simulink model "Bdot"  (R2023b)
settings: Solver=VariableStepAuto  StartTime=0.0  StopTime=2.647E4  FixedStep=1  MaxStep=100  RelTol=1e-3
model workspace (MAT data in the model file):
  Inertia = [0.0088  0  0; 0  0.0088  0; 0  0  0.004]
  M = 0.9
  T = 5580
libraries: matrix_library x2, shared6dof x1, simulink x1, aerolibanim x1
settings Model: Creator=bogas  LastModifiedBy=bogas

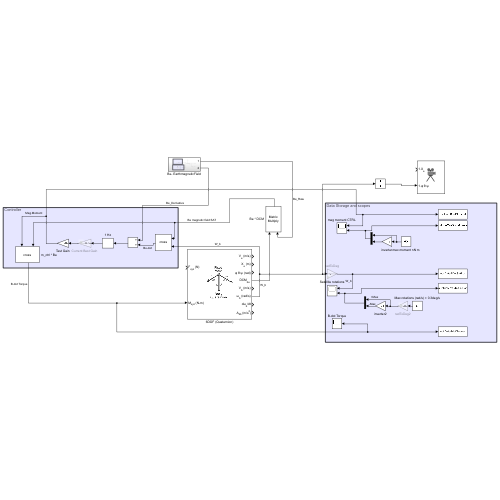
[thumbnail: Simulink's stored preview of the top-level diagram]
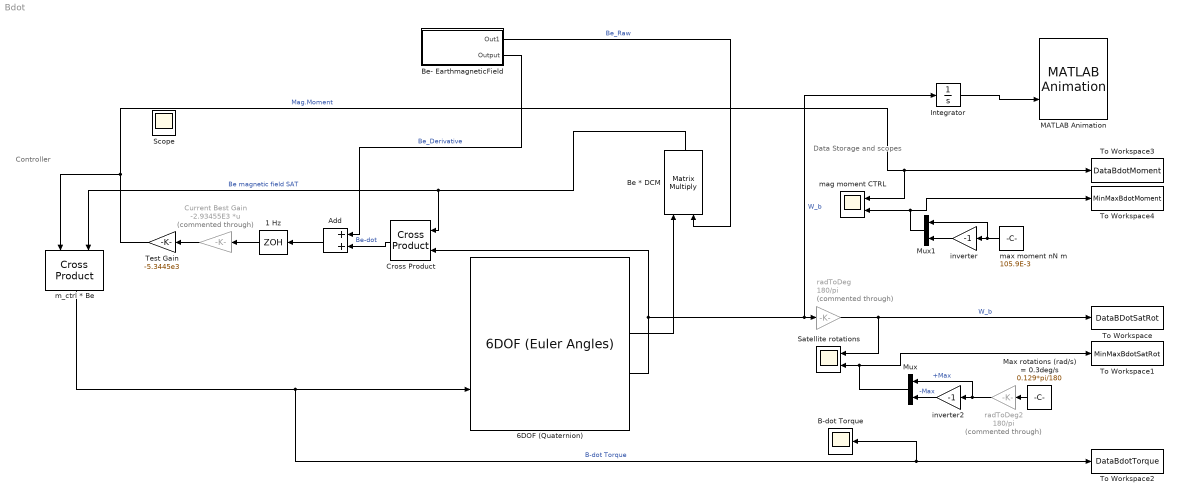
== system Bdot ==
  note: Controller
  note: Data Storage and scopes
  1 Hz : ZeroOrderHold
  6DOF (Quaternion) : shared6dof/6DOF (Euler Angles)  units=Metric (MKS)  mtype=Fixed  rep=Quaternion  xme_0=[0 0 0]  Vm_0=[0 0 0]  eul_0=[0 0 0]  pm_0=0.1745*[1,1,1]  mass_0=M  mass_e=0.5  mass_f=2.0  inertia=Inertia  inertia_e=eye(3)  inertia_f=2*eye(3)  k_quat=1.0  vre_flag=on  abi_flag=off  aMode=0  xme_statename=''  Vm_statename=''  eul_statename=''  quat_statename=''  pm_statename=''  mass_statename=''
      settings: LibrarySourceBlock=aerolib6dof2/6DOF (Quaternion)
  Add : Sum
  B-dot Torque : Scope
  Be * DCM : Product  Multiplication=Matrix(*)
  Be- EarthmagneticField : Subsystem
  Cross Product : matrix_library/Cross Product
  Current Best Gain : Gain  Commented=through  Gain=-2.93455E3  Multiplication=Matrix(K*u)
  Integrator : Integrator
  MATLAB Animation : aerolibanim/MATLAB Animation  Tag=Matlab Animation 6 DOF  Vehicles=1  Geometries='astredwedge.mat'  BoundingBoxCoordinates=[-50,50,-50,50,-50,50]  CameraOffset=[-150,-50,0]  CameraViewAngle=3  SampleTime=10  FigurePosition=[962,50,958,973]
  Max rotations (rad/s) = 0.3deg/s : Constant  Value=0.129*pi/180
  Mux : Mux  Inputs=2
  Mux1 : Mux  Inputs=2
  Satellite rotations : Scope  NumInputPorts=2
  Test Gain : Gain  Gain=-5.3445e3
  To Workspace : ToWorkspace  VariableName=DataBDotSatRot  SaveFormat=Timeseries  SampleTime=-1
  To Workspace1 : ToWorkspace  VariableName=MinMaxBdotSatRot  SaveFormat=Timeseries  SampleTime=-1
  To Workspace2 : ToWorkspace  VariableName=DataBdotTorque  SaveFormat=Timeseries  SampleTime=-1
  To Workspace3 : ToWorkspace  VariableName=DataBdotMoment  SaveFormat=Timeseries  SampleTime=-1
  To Workspace4 : ToWorkspace  VariableName=MinMaxBdotMoment  SaveFormat=Timeseries  SampleTime=-1
  inverter : Gain  Gain=-1
  inverter2 : Gain  Gain=-1
  m_ctrl * Be : matrix_library/Cross Product
  mag moment CTRL : Scope  NumInputPorts=2
  max moment nN m : Constant  Value=105.9E-3
  radToDeg : Gain  Commented=through  Gain=180/pi
  radToDeg2 : Gain  Commented=through  Gain=180/pi
  Scope : Scope
  wires:
  6DOF (Quaternion)/6 -> Cross Product/2, Integrator/1, radToDeg/1  "W_b"
  Be * DCM/1 -> Cross Product/1, m_ctrl * Be/2  "Be magnetic field SAT"
  Test Gain/1 -> m_ctrl * Be/1, mag moment CTRL/1, To Workspace3/1  "Mag.Moment"
  m_ctrl * Be/1 -> To Workspace2/1, B-dot Torque/1, 6DOF (Quaternion)/2  "B-dot Torque"
  6DOF (Quaternion)/4 -> Be * DCM/1
  max moment nN m/1 -> inverter/1, Mux1/1
  1 Hz/1 -> Current Best Gain/1
  Max rotations (rad/s) = 0.3deg/s/1 -> radToDeg2/1
  inverter2/1 -> Mux/2  "-Max"
  Mux/1 -> To Workspace1/1, Satellite rotations/2
  Mux1/1 -> To Workspace4/1, mag moment CTRL/2
  inverter/1 -> Mux1/2
  Be- EarthmagneticField/1(Out1) -> Be * DCM/2  "Be_Raw"
  Be- EarthmagneticField/2(Output) -> Add/1  "Be_Derivative"
  Add/1 -> 1 Hz/1
  Cross Product/1 -> Add/2  "Be-dot"
  radToDeg/1 -> To Workspace/1, Satellite rotations/1  "W_b"
  radToDeg2/1 -> Mux/1, inverter2/1  "+Max"
  Current Best Gain/1 -> Test Gain/1
  Integrator/1 -> MATLAB Animation/2

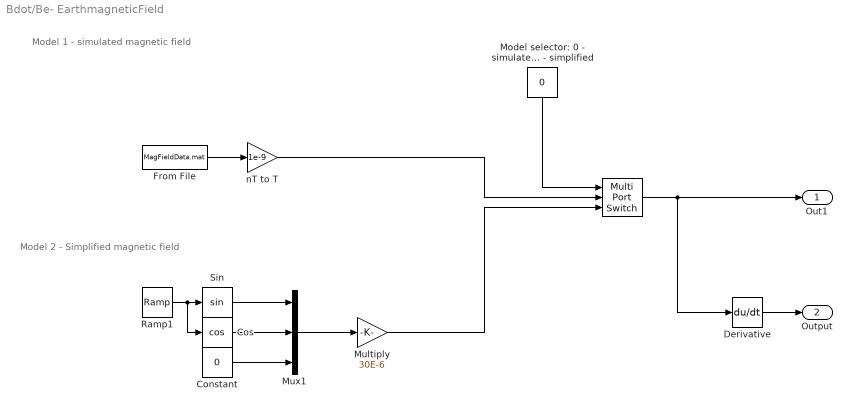
== system Bdot/Be- EarthmagneticField ==
  note: Model 2 - Simplified magnetic field
  note: Model 1 - simulated magnetic field
  " " : MultiPortSwitch  DataPortOrder=Zero-based contiguous  Inputs=2  zeroidx=on  OutMin=[0]  OutMax=[26470]  SaturateOnIntegerOverflow=off  InputSameDT=off
  Constant : Constant  Value=0
  Cos : Trigonometry  Operator=cos
  Derivative : Derivative
  From File : FromFile  FileName=MagFieldData.mat  SampleTime=0
  "Model selector: 0 - simulated 1 - simplified " : Constant  Value=0
  Multiply : Gain  Gain=30E-6
  Mux1 : Mux  Inputs=3
  Ramp1 : simulink/Sources/Ramp  slope=2*pi/T  start=0  InitialOutput=0
  Sin : Trigonometry
  nT to T : Gain  Gain=1e-9
  Out1 : Outport
  Output : Outport  Port=2
  wires:
  Derivative/1 -> Output/1
  Mux1/1 -> Multiply/1
  Ramp1/1 -> Cos/1, Sin/1
  Cos/1 -> Mux1/2
  Sin/1 -> Mux1/1
  Constant/1 -> Mux1/3
  From File/1 -> nT to T/1
  "Model selector: 0 - simulated 1 - simplified "/1 -> " "/1
  " "/1 -> Derivative/1, Out1/1
  nT to T/1 -> " "/2
  Multiply/1 -> " "/3
